simulink model "EKF_sim"  (R2021a)
settings: Solver=ode45  StartTime=0.0  StopTime=450  MaxStep=0.1  RelTol=1e-3  EnableMultiTasking=on
model workspace (MATLAB code in the model file + MAT data in the model file):
  L = 2.5
  v0 = 0
  xe0 = 0
  xn0 = 0
  theta0 = 0
  Ts = 1
  rr = [0 0 0 0 0 0 0 0 0 0 0 0 ... (9404 elements, 9404x1)]
  tt = [0 0.05 0.1 0.15 0.2 0.25 0.3 0.35 0.4 0.45 0.5 0.55 ... (9404 elements, 9404x1)]
  vv = [25 25 25 25 25 25 25 25 25 25 25 25 ... (9404 elements, 9404x1)]
libraries: simulink x2, pid_lib x2, sharedTrackingLibrary x1
(part 2 of 2)

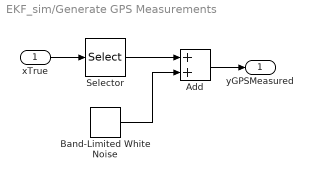
== system EKF_sim/Generate GPS Measurements ==
  xTrue : Inport  SampleTime=20*Ts
  Add : Sum
  Band-Limited White Noise : simulink/Sources/Band-Limited White Noise  Cov=50  Ts=1  seed=[23343;23344]
  Selector : Selector  InputPortWidth=4  IndexOptions=Index vector (dialog)  Indices=[1:2]  OutputSizes=1
  yGPSMeasured : Outport  VectorParamsAs1DForOutWhenUnconnected=off
  wires:
  xTrue/1 -> Selector/1
  Selector/1 -> Add/1
  Add/1 -> yGPSMeasured/1
  Band-Limited White Noise/1 -> Add/2

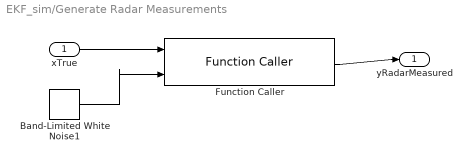
== system EKF_sim/Generate Radar Measurements ==
  xTrue : Inport  SampleTime=0.05
  Band-Limited White Noise1 : simulink/Sources/Band-Limited White Noise  Cov=5e-5  Ts=1  seed=[23341;23342]
  Function Caller : FunctionCaller  FunctionPrototype=y = radarMeasurementFcn(x,v)  InputArgumentSpecifications=zeros(4,1), zeros(2,1)  OutputArgumentSpecifications=zeros(2,1)
  yRadarMeasured : Outport  VectorParamsAs1DForOutWhenUnconnected=off
  wires:
  Function Caller/1 -> yRadarMeasured/1
  xTrue/1 -> Function Caller/1
  Band-Limited White Noise1/1 -> Function Caller/2

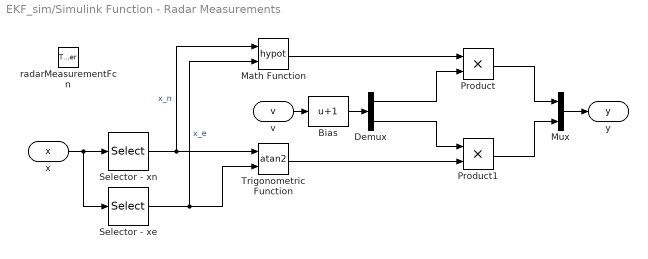
== system EKF_sim/Simulink Function - Radar Measurements ==
  radarMeasurementFcn : TriggerPort  TriggerType=function-call  IsSimulinkFunction=on  FunctionName=radarMeasurementFcn  VariantControl=Variant
  Bias : Bias  Bias=1
  Demux : Demux  Outputs=2
  Math Function : Math  Operator=hypot  SignedPower=on  SaturateOnIntegerOverflow=on
  Mux : Mux  Inputs=2
  Product : Product
  Product1 : Product
  Selector - xe : Selector  InputPortWidth=4  IndexOptions=Index vector (dialog)  Indices=1  OutputSizes=1
  Selector - xn : Selector  InputPortWidth=4  IndexOptions=Index vector (dialog)  Indices=2  OutputSizes=1
  Trigonometric Function : Trigonometry  Operator=atan2
  x : ArgIn  DisableCoverage=on  PortDimensions=4  ArgumentName=x
  v : ArgIn  DisableCoverage=on  Port=2  PortDimensions=2  ArgumentName=v
  y : ArgOut  DisableCoverage=on  PortDimensions=2  ArgumentName=y
  wires:
  Mux/1 -> y/1
  x/1 -> Selector - xe/1, Selector - xn/1
  Selector - xn/1 -> Math Function/1, Trigonometric Function/1  "x_n"
  Selector - xe/1 -> Math Function/2, Trigonometric Function/2  "x_e"
  Trigonometric Function/1 -> Product1/2
  v/1 -> Bias/1
  Math Function/1 -> Product/1
  Product/1 -> Mux/1
  Product1/1 -> Mux/2
  Bias/1 -> Demux/1
  Demux/1 -> Product/2
  Demux/2 -> Product1/1

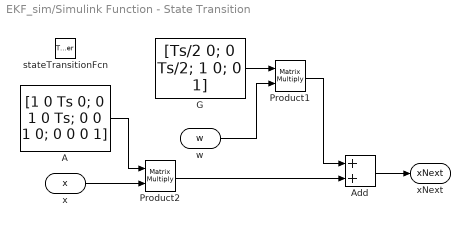
== system EKF_sim/Simulink Function - State Transition ==
  stateTransitionFcn : TriggerPort  TriggerType=function-call  IsSimulinkFunction=on  FunctionName=stateTransitionFcn  VariantControl=Variant
  A : Constant  Value=[1 0 Ts 0; 0 1 0 Ts; 0 0 1 0; 0 0 0 1]
  Add : Sum
  G : Constant  Value=[Ts/2 0; 0 Ts/2; 1 0; 0 1]
  Product1 : Product  Multiplication=Matrix(*)
  Product2 : Product  Multiplication=Matrix(*)
  x : ArgIn  DisableCoverage=on  PortDimensions=4  ArgumentName=x
  w : ArgIn  Port=2  PortDimensions=2  ArgumentName=w
  xNext : ArgOut  DisableCoverage=on  PortDimensions=4  ArgumentName=xNext
  wires:
  x/1 -> Product2/2
  A/1 -> Product2/1
  Product2/1 -> Add/2
  G/1 -> Product1/1
  w/1 -> Product1/2
  Product1/1 -> Add/1
  Add/1 -> xNext/1

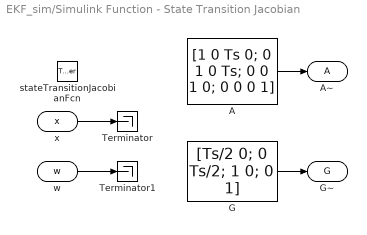
== system EKF_sim/Simulink Function - State Transition Jacobian ==
  stateTransitionJacobianFcn : TriggerPort  TriggerType=function-call  IsSimulinkFunction=on  FunctionName=stateTransitionJacobianFcn  VariantControl=Variant
  A : Constant  Value=[1 0 Ts 0; 0 1 0 Ts; 0 0 1 0; 0 0 0 1]
  G : Constant  Value=[Ts/2 0; 0 Ts/2; 1 0; 0 1]
  Terminator : Terminator
  Terminator1 : Terminator
  x : ArgIn  DisableCoverage=on  PortDimensions=4  ArgumentName=x
  w : ArgIn  Port=2  PortDimensions=2  ArgumentName=w
  A~ : ArgOut  DisableCoverage=on  PortDimensions=[4 4]  ArgumentName=A
  G~ : ArgOut  Port=2  PortDimensions=[4 2]  ArgumentName=G
  wires:
  G/1 -> G~/1
  x/1 -> Terminator/1
  w/1 -> Terminator1/1
  A/1 -> A~/1

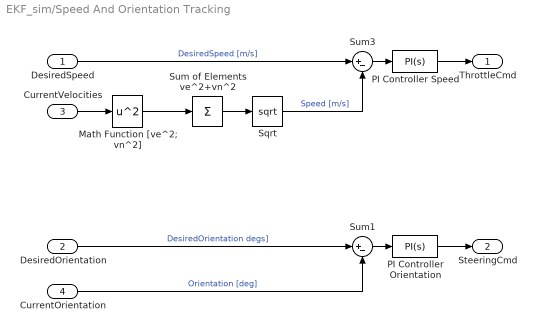
== system EKF_sim/Speed And Orientation Tracking ==
  DesiredSpeed : Inport
  DesiredOrientation : Inport  Port=2
  CurrentVelocities : Inport  Port=3
  CurrentOrientation : Inport  Port=4
  Math Function [ve^2; vn^2] : Math  Operator=square  SignedPower=on  SaturateOnIntegerOverflow=on
  PI Controller Orientation : pid_lib/PID Controller  Controller=PI  Form=Parallel  TimeDomain=Continuous-time  UseExternalTs=off  SampleTime=-1  IntegratorMethod=Forward Euler  FilterMethod=Forward Euler  ControllerParametersSource=internal  P=1  I=0.3  D=0  UseFilter=on  N=100  TunerSelectOption=Transfer Function Based (PID Tuner App)  InitialConditionSource=internal  InitialConditionForIntegrator=0  InitialConditionForFilter=0  DifferentiatorICPrevScaledInput=0  ExternalReset=none  TrackingMode=off  Kt=1  LimitOutput=on  SatLimitsSource=internal  UpperSaturationLimit=20  LowerSaturationLimit=-20  LinearizeAsGain=off  AntiWindupMode=clamping  Kb=1  POutMin=[]  POutMax=[]  IOutMin=[]  IOutMax=[]  DOutMin=[]  DOutMax=[]  NOutMin=[]  NOutMax=[]  SumOutMin=[]  SumOutMax=[]  SaturationOutMin=[]  SaturationOutMax=[]  PParamMin=[]  PParamMax=[]  IParamMin=[]  IParamMax=[]  DParamMin=[]  DParamMax=[]  NParamMin=[]  NParamMax=[]  KbParamMin=[]  KbParamMax=[]  KtParamMin=[]  KtParamMax=[]  KbOutMin=[]  KbOutMax=[]  KtOutMin=[]  KtOutMax=[]  IntegratorOutMin=[]  IntegratorOutMax=[]  FilterOutMin=[]  FilterOutMax=[]  SumI1OutMin=[]  SumI1OutMax=[]  SumI2OutMin=[]  SumI2OutMax=[]  SumI3OutMin=[]  SumI3OutMax=[]  SumI4OutMin=[]  SumI4OutMax=[]  SumDOutMin=[]  SumDOutMax=[]  DifferentiatorOutMin=[]  DifferentiatorOutMax=[]  FilterDiffOutCoefMin=[]  FilterDiffOutCoefMax=[]  ReciprocalOutMin=[]  ReciprocalOutMax=[]  SumDenOutMin=[]  SumDenOutMax=[]  SumNumOutMin=[]  SumNumOutMax=[]  DivideOutMin=[]  DivideOutMax=[]  UdiffTsProdOutMin=[]  UdiffTsProdOutMax=[]  NTsProdOutMin=[]  NTsProdOutMax=[]  UintegralTsProdOutMin=[]  UintegralTsProdOutMax=[]  UngainTsProdOutMin=[]  UngainTsProdOutMax=[]  IntegratorContinuousStateAttributes=''  IntegratorStateMustResolveToSignalObject=off  IntegratorRTWStateStorageClass=Auto  FilterContinuousStateAttributes=''  FilterStateMustResolveToSignalObject=off  FilterRTWStateStorageClass=Auto  ParallelPVariant=InternalParameters  IdealPVariant=Disabled  IVariant=InternalParameters  DVariant=Disabled  IntegratorVariant=Continuous  SatVariant=Enabled  AWVariant=ContClampingParallel  PCopyVariant=Disabled  TRVariant=Disabled  FdbkBlocksVariant=Forward  IdealPFdbkVariant=Disabled  SatFdbkVariant=Disabled  DerivativeFilterVariant=Disabled  NVariant=Disabled  NCopyVariant=Disabled_SignalSpec  FilterICVariant=Disabled  IntegratorICVariant=InternalICs  ExternalResetVariant=Disabled  TRSumVariant=Passthrough  SumFdbkVariant=Disabled  SumVariant=Sum_PI  TsampFilterVariant=InternalTs  TsampNgainVariant=Passthrough  TsampIntegralVariant=Passthrough  ExternalSaturationOutDataTypeStr=Inherit: Same as second input
  PI Controller Speed : pid_lib/PID Controller  Controller=PI  Form=Parallel  TimeDomain=Continuous-time  UseExternalTs=off  SampleTime=-1  IntegratorMethod=Forward Euler  FilterMethod=Forward Euler  ControllerParametersSource=internal  P=0.15  I=0.01  D=0  UseFilter=on  N=100  TunerSelectOption=Transfer Function Based (PID Tuner App)  InitialConditionSource=internal  InitialConditionForIntegrator=0  InitialConditionForFilter=0  DifferentiatorICPrevScaledInput=0  ExternalReset=none  TrackingMode=off  Kt=1  LimitOutput=on  SatLimitsSource=internal  UpperSaturationLimit=1  LowerSaturationLimit=-1  LinearizeAsGain=off  AntiWindupMode=clamping  Kb=1  POutMin=[]  POutMax=[]  IOutMin=[]  IOutMax=[]  DOutMin=[]  DOutMax=[]  NOutMin=[]  NOutMax=[]  SumOutMin=[]  SumOutMax=[]  SaturationOutMin=[]  SaturationOutMax=[]  PParamMin=[]  PParamMax=[]  IParamMin=[]  IParamMax=[]  DParamMin=[]  DParamMax=[]  NParamMin=[]  NParamMax=[]  KbParamMin=[]  KbParamMax=[]  KtParamMin=[]  KtParamMax=[]  KbOutMin=[]  KbOutMax=[]  KtOutMin=[]  KtOutMax=[]  IntegratorOutMin=[]  IntegratorOutMax=[]  FilterOutMin=[]  FilterOutMax=[]  SumI1OutMin=[]  SumI1OutMax=[]  SumI2OutMin=[]  SumI2OutMax=[]  SumI3OutMin=[]  SumI3OutMax=[]  SumI4OutMin=[]  SumI4OutMax=[]  SumDOutMin=[]  SumDOutMax=[]  DifferentiatorOutMin=[]  DifferentiatorOutMax=[]  FilterDiffOutCoefMin=[]  FilterDiffOutCoefMax=[]  ReciprocalOutMin=[]  ReciprocalOutMax=[]  SumDenOutMin=[]  SumDenOutMax=[]  SumNumOutMin=[]  SumNumOutMax=[]  DivideOutMin=[]  DivideOutMax=[]  UdiffTsProdOutMin=[]  UdiffTsProdOutMax=[]  NTsProdOutMin=[]  NTsProdOutMax=[]  UintegralTsProdOutMin=[]  UintegralTsProdOutMax=[]  UngainTsProdOutMin=[]  UngainTsProdOutMax=[]  IntegratorContinuousStateAttributes=''  IntegratorStateMustResolveToSignalObject=off  IntegratorRTWStateStorageClass=Auto  FilterContinuousStateAttributes=''  FilterStateMustResolveToSignalObject=off  FilterRTWStateStorageClass=Auto  ParallelPVariant=InternalParameters  IdealPVariant=Disabled  IVariant=InternalParameters  DVariant=Disabled  IntegratorVariant=Continuous  SatVariant=Enabled  AWVariant=ContClampingParallel  PCopyVariant=Disabled  TRVariant=Disabled  FdbkBlocksVariant=Forward  IdealPFdbkVariant=Disabled  SatFdbkVariant=Disabled  DerivativeFilterVariant=Disabled  NVariant=Disabled  NCopyVariant=Disabled_SignalSpec  FilterICVariant=Disabled  IntegratorICVariant=InternalICs  ExternalResetVariant=Disabled  TRSumVariant=Passthrough  SumFdbkVariant=Disabled  SumVariant=Sum_PI  TsampFilterVariant=InternalTs  TsampNgainVariant=Passthrough  TsampIntegralVariant=Passthrough  ExternalSaturationOutDataTypeStr=Inherit: Same as second input
  Sqrt : Sqrt  SaturateOnIntegerOverflow=on
  Sum of Elements ve^2+vn^2 : Sum  Inputs=+
  Sum1 : Sum  Inputs=|+-
  Sum3 : Sum  Inputs=|+-
  ThrottleCmd : Outport
  SteeringCmd : Outport  Port=2
  wires:
  PI Controller Speed/1 -> ThrottleCmd/1
  DesiredSpeed/1 -> Sum3/1  "DesiredSpeed [m/s]"
  Sum3/1 -> PI Controller Speed/1
  CurrentVelocities/1 -> Math Function [ve^2; vn^2]/1
  Math Function [ve^2; vn^2]/1 -> Sum of Elements ve^2+vn^2/1
  Sum of Elements ve^2+vn^2/1 -> Sqrt/1
  Sqrt/1 -> Sum3/2  "Speed [m/s]"
  PI Controller Orientation/1 -> SteeringCmd/1
  DesiredOrientation/1 -> Sum1/1  "DesiredOrientation degs]"
  Sum1/1 -> PI Controller Orientation/1
  CurrentOrientation/1 -> Sum1/2  "Orientation [deg]"

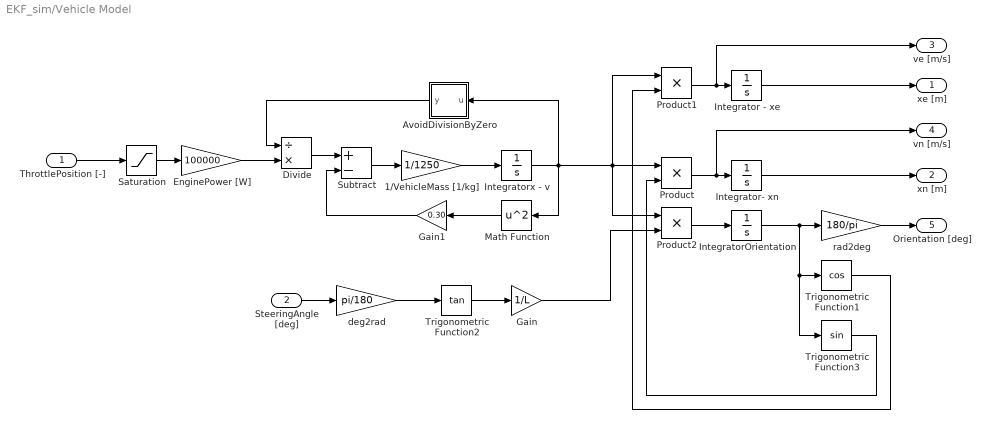
== system EKF_sim/Vehicle Model ==
  ThrottlePosition [-] : Inport
  "SteeringAngle [deg] " : Inport  Port=2
  1/VehicleMass [1/kg] : Gain  Gain=1/1250
  AvoidDivisionByZero : Subsystem
  Divide : Product  Inputs=/*
  EnginePower [W] : Gain  Gain=100000
  Gain : Gain  Gain=1/L
  Gain1 : Gain  Gain=0.30
  Integrator - xe : Integrator  InitialCondition=xe0
  Integrator- xn : Integrator  InitialCondition=xn0
  IntegratorOrientation : Integrator  InitialCondition=theta0
  Integratorx - v : Integrator  InitialCondition=v0
  Math Function : Math  Operator=square  SignedPower=on  SaturateOnIntegerOverflow=on
  Product : Product
  Product1 : Product
  Product2 : Product
  Saturation : Saturate  UpperLimit=1  LowerLimit=-1
  Subtract : Sum  Inputs=+-
  Trigonometric Function1 : Trigonometry  Operator=cos
  Trigonometric Function2 : Trigonometry  Operator=tan
  Trigonometric Function3 : Trigonometry
  deg2rad : Gain  Gain=pi/180
  rad2deg : Gain  Gain=180/pi
  xe [m] : Outport
  xn [m] : Outport  Port=2
  ve [m/s] : Outport  Port=3
  vn [m/s] : Outport  Port=4
  Orientation [deg] : Outport  Port=5
  wires:
  Trigonometric Function3/1 -> Product/2
  Product/1 -> vn [m/s]/1, Integrator- xn/1
  Product1/1 -> ve [m/s]/1, Integrator - xe/1
  Product2/1 -> IntegratorOrientation/1
  "SteeringAngle [deg] "/1 -> deg2rad/1
  Gain/1 -> Product2/2
  Trigonometric Function2/1 -> Gain/1
  Integrator - xe/1 -> xe [m]/1
  Integrator- xn/1 -> xn [m]/1
  IntegratorOrientation/1 -> Trigonometric Function3/1, Trigonometric Function1/1, rad2deg/1
  deg2rad/1 -> Trigonometric Function2/1
  rad2deg/1 -> Orientation [deg]/1
  ThrottlePosition [-]/1 -> Saturation/1
  Integratorx - v/1 -> Math Function/1, AvoidDivisionByZero/1(u), Product1/1, Product/1, Product2/1
  Saturation/1 -> EnginePower [W]/1
  EnginePower [W]/1 -> Divide/2
  AvoidDivisionByZero/1(y) -> Divide/1
  Trigonometric Function1/1 -> Product1/2
  Divide/1 -> Subtract/1
  Subtract/1 -> 1/VehicleMass [1/kg]/1
  Math Function/1 -> Gain1/1
  Gain1/1 -> Subtract/2
  1/VehicleMass [1/kg]/1 -> Integratorx - v/1

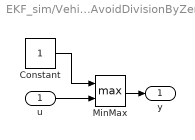
== system EKF_sim/Vehicle Model/AvoidDivisionByZero ==
  u : Inport
  Constant : Constant
  MinMax : MinMax  Function=max  Inputs=2
  y : Outport
  wires:
  MinMax/1 -> y/1
  Constant/1 -> MinMax/1
  u/1 -> MinMax/2
